simulink model "Bands5"  (R2018a)
settings: Solver=VariableStepAuto  StartTime=0.0  StopTime=0.01  RelTol=1e-3
undefined symbols (not defined in the file): fdesignblkfcn, G1, G2, G3, G4, G5, gcbh, get, T
libraries: dspsrcs4 x1, dspxfrm3 x1, dspobslib x1
(part 2 of 2)

== system Bands5/Filter Bank /Filter 5/Bandpass Filter ==
  In : Inport
  Generated Filter Block : DiscreteFir  Tag=BlockMethodSubSystem  Coefficients=[-1.37477644203245411e-07 1.09856442472417534e-06 -4.41572652330620209e-06 1.21444897004689071e-05 -2.50073620655742345e-05 3.92878095826258104e-05 -4.4547465686985446e-05 2.58949291023641021e-05 2.65953520742472641e-05 -0.000103788029815876713 0.000168285176535554599 -0.000162957657537141006 4.32347953880678207e-05 0.00017831490456862427 -0.000405265451320053246 0.000481931728292018548 -0.000278594346697857553 -0.000198731661938878797 0.000748379970081961888 -0.00103259053796100051 0.000762687981402191675 7.90106887629365138e-05 -0.00113169662266953178 0.0017816099019439635 -0.00150455227629922757 0.000244094729826234912 0.00143343040340180639 -0.00257224318819057433 0.00237481568040012834 -0.000750116391036459397 -0.0015140061025354886 0.00313395596656663262 -0.00308967391539442153 0.00129493525261987607 0.00128038138881878894 -0.00316369450845424213 0.00328267047898157371 -0.00163145258283516796 -0.000749151773731452806 0.00246603969592711515 -0.00266468783836855926 0.00150617386989928561 7.30064054535404101e-05 -0.00109734205224688202 0.0012144255103374987 -0.000802045690174915302 0.000495187029089933601 -0.00056812830028998818 0.000704378614726650521 -0.000344487811539014737 -0.000699788879420734926 0.00191959201810252655 -0.00239947898650042348 0.00153339911544199989 0.000407701875158527412 -0.0023478363793530293 0.00311083668377376901 -0.00223820333079517318 0.000295537163000701871 0.00155872958527764191 -0.00238984222654471928 0.00205090890795089215 -0.00109557446152876072 0.000192385455316903587 0.000411167237244330452 -0.00092046515735622037 0.00155386209107931383 -0.00210549157266725403 0.00198412065253432239 -0.000752478880387533601 -0.00130517037093062825 0.00314752030705167706 -0.00360804523600666976 0.00224487124711793577 0.000272090935558694702 -0.00257466850450670899 0.00350674618685953201 -0.00283016287963893786 0.00121196124101988992 0.000414209674220371771 -0.00152103904436424954 0.00214084343489315092 -0.00246684891893655337 0.00239082020924767744 -0.00150454838029059922 -0.000386756826904268293 0.0027414036505342531 -0.00434239107851502708 0.00404911338529099704 -0.00169688039219482219 -0.00161461801539797669 0.0041547621325787364 -0.00467631169637095032 0.00316327385870383707 -0.000667703777904009939 -0.00155436321326024238 0.00284904353002525318 -0.00328570068970270848 0.00313930148243870633 -0.00236730486372858538 0.00067045215976253012 0.00190333696579673452 -0.00446649908567267953 0.00555486712302272548 -0.00411873084223472047 0.000477992732617617234 0.00362383865710449917 -0.00604586024150340247 0.00562870864189406531 -0.00287200191055806894 -0.000579800898621379889 0.00315614445904127032 -0.00426122185575505096 0.00420404674351268926 -0.00342602439464845645 0.00191219742444212817 0.00058419825636181076 -0.00375604122683084784 0.0063029187831130434 -0.00651061843443168434 0.0035631857403312611 0.00150370549017589438 -0.00615609852227420786 0.00792476147302343011 -0.00602608314871479461 0.00177891197411728054 0.00247094916378937622 -0.00498421263043891984 0.00548980200436181062 -0.00471826562518968227 0.00327410957941588624 -0.00105780864127851004 -0.00218783219630085211 0.00583775818597942302 -0.00808748654065121614 0.00700767601350604352 -0.00223093913183317061 -0.00423254655145381773 0.00898215801929982266 -0.00943888294084165025 0.00558348709224518354 0.000166017052079085259 -0.00479643066112162789 0.00670531152682119023 -0.00627186769717235758 0.00475233779712449633 -0.00277073249214325468 -5.52515908403549571e-05 0.00403111147752428789 -0.00806745489575687487 0.00971605950987917966 -0.00691244581249528863 4.30783488861863424e-05 0.00761869872667154079 -0.011818881648909263 0.0102410703051660414 -0.0041063207071181055 -0.00285938146877273529 0.00720236771192633764 -0.00793300710571490965 0.0064201869258872753 -0.0043983533257234567 0.00217509750490524865 0.00119438573282819316 -0.0060234324930620092 0.0104640325660529162 -0.0112090524765636225 0.00619723117819840404 0.00300772009442789494 ...(+7136 chars)]  InputProcessing=Columns as channels (frame based)
  Out : Outport
  wires:
  In/1 -> Generated Filter Block/1
  Generated Filter Block/1 -> Out/1
